simulink model "lab12"  (Simulink 8.5)
settings: Solver=ode45  StartTime=0.0  StopTime=1000000  RelTol=1e-3
settings Model: Creator=Meteo  LastModifiedBy=Meteo
settings DataIOCC: SignalLoggingSaveFormat=Dataset
settings OptimizationCC: ExpressionDepthLimit=128
settings DebuggingCC: UnderspecifiedInitializationDetection=Simplified  MergeDetectMultiDrivingBlocksExec=error  FcnCallInpInsideContextMsg=EnableAllAsError  StateNameClashWarn=none
settings GRTTargetCC: CombineOutputUpdateFcns=on  GRTInterface=off
settings SimEventsCC: propDiagStatOutput=0

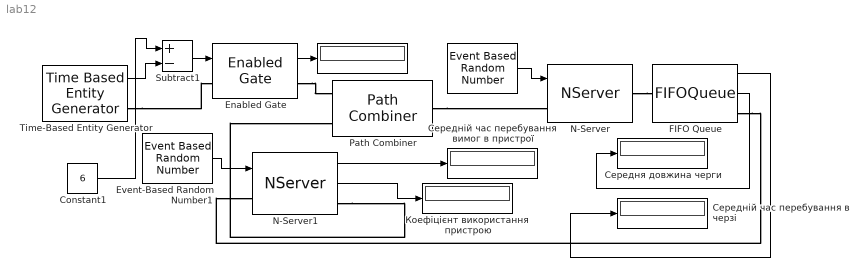
== system lab12 ==
  " " : EventBasedRandomNumber  Distribution=Poisson  meanExp=27  meanPoiss=27
  "   " : Display
  Constant1 : Constant  Value=6
  Enabled Gate : EnabledGate  SpecifyEventPriority=on  StatNumberDeparted=on
  Event-Based Random Number1 : EventBasedRandomNumber  meanExp=17  meanPoiss=17
  FIFO Queue : FIFOQueue  Capacity=4  StatAverageWait=on  StatAverageQueueLength=on
      settings: OutputPortMap=o2,o3
  N-Server : NServer  NumberOfServers=6  ServiceTimeFrom=Signal port t
  N-Server1 : NServer  NumberOfServers=2  ServiceTimeFrom=Signal port t  StatAverageWait=on  StatUtilization=on
      settings: OutputPortMap=o4,o5
  Path Combiner : PathCombiner  NumberInputPorts=2
  Subtract1 : Sum  Inputs=+-
  Time-Based Entity Generator : TimeBasedEntityGenerator  Distribution=Exponential  Period=34  InitialSeed=61357  Mean=27  StatNumberDeparted=on
  Коефіцієнт використання  пристрою : Display
  Середня довжина черги : Display
  Середній час перебування  вимог в пристрої : Display
  Середній час перебування в черзі : Display
  wires:
  FIFO Queue/2 -> Середня довжина черги/1
  " "/1 -> N-Server/1
  FIFO Queue/1 -> Середній час перебування в черзі/1
  Subtract1/1 -> Enabled Gate/1
  Time-Based Entity Generator/1 -> Subtract1/2
  Enabled Gate/1 -> "   "/1
  Constant1/1 -> Subtract1/1
  N-Server1/2 -> Коефіцієнт використання  пристрою/1
  N-Server1/1 -> Середній час перебування  вимог в пристрої/1
  Event-Based Random Number1/1 -> N-Server1/1
  connections:
  Time-Based Entity Generator/RConn1 -- Enabled Gate/LConn1
  Enabled Gate/RConn1 -- Path Combiner/LConn1
  N-Server1/RConn1 -- Path Combiner/LConn2
  Path Combiner/RConn1 -- N-Server/LConn1
  N-Server/RConn1 -- FIFO Queue/LConn1
  FIFO Queue/RConn1 -- N-Server1/LConn1
